simulink model "H_f_Greska_inverzna_staticka_karakteristika"  (R2016a)
settings: Solver=VariableStepAuto  StartTime=0.0  StopTime=800  RelTol=1e-3
undefined symbols (not defined in the file): ln
libraries: simulink x2
settings Model: Creator=AmelT  LastModifiedBy=AmelT

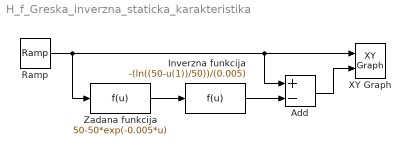
== system H_f_Greska_inverzna_staticka_karakteristika ==
  Add : Sum  Inputs=+-
  Inverzna funkcija : Fcn  Expr=-(ln((50-u(1))/50))/(0.005)
  Ramp : simulink/Sources/Ramp  slope=1  start=0  X0=0
  XY Graph : simulink/Sinks/XY Graph  xmin=0  xmax=800  ymin=-0.01  ymax=0.01  st=1
  Zadana funkcija : Fcn  Expr=50-50*exp(-0.005*u)
  wires:
  Zadana funkcija/1 -> Inverzna funkcija/1
  Ramp/1 -> Zadana funkcija/1, Add/1, XY Graph/1
  Inverzna funkcija/1 -> Add/2
  Add/1 -> XY Graph/2
